simulink model "Crazyflie_NoLinealModel_EB"  (R2020b)
settings: Solver=FixedStepAuto  StartTime=0.0  StopTime=30  FixedStep=0.001  RelTol=1e-3
values from neighbouring files (symbols this model uses):
  fm = 0.2685    [Crazyflie_Model.m]
  we = sqrt((m*g)/(4*CT))    [Crazyflie_Model.m]
undefined symbols (not defined in the file or in its folder): DiscIntNeverNeededParam, Dphi_s, Dphi_T, Dpsi_s, Dtheta_s, KIz, magnitude, MCO, Phi_s, Phi_T, phi_theta_limit, quad, Theta_s, U_s, V_s, X_s, X_T, XY_delta, xyv_lim, Y_s, Yaw_delta, Yaw_s, Yaw_T, Z_delta, Z_s, Z_T
libraries: simulink x16, pid_lib x11
(part 2 of 2)

== system Crazyflie_NoLinealModel_EB/On-board Controllers/Control Mixer ==
  OMEGA : Inport
  Dpitch : Inport  Port=2
  Droll : Inport  Port=3
  Dyaw : Inport  Port=4
  Enable : EnablePort
  Demux : Demux
  Gain : Gain  Gain=MCO  Multiplication=Matrix(K*u) (u vector)
  Mux : Mux
  PWM1 : Outport
  PWM2 : Outport  Port=2
  PWM3 : Outport  Port=3
  PWM4 : Outport  Port=4
  wires:
  Mux/1 -> Gain/1
  Gain/1 -> Demux/1
  Demux/3 -> PWM3/1
  Demux/1 -> PWM1/1
  Demux/2 -> PWM2/1
  Droll/1 -> Mux/3
  OMEGA/1 -> Mux/1
  Dyaw/1 -> Mux/4
  Dpitch/1 -> Mux/2
  Demux/4 -> PWM4/1

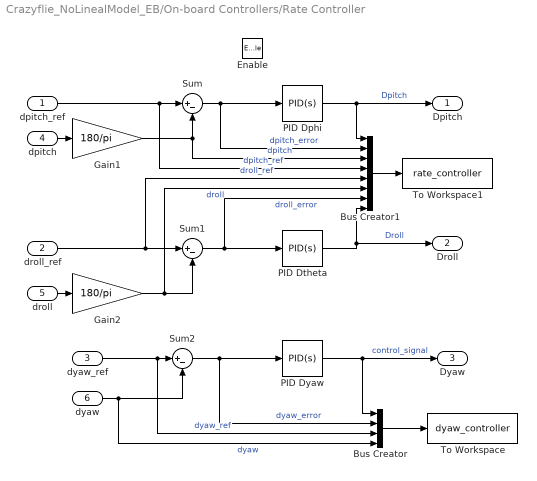
== system Crazyflie_NoLinealModel_EB/On-board Controllers/Rate Controller ==
  dpitch_ref : Inport
  droll_ref : Inport  Port=2
  dyaw_ref : Inport  Port=3
  dpitch : Inport  Port=4
  droll : Inport  Port=5
  dyaw : Inport  Port=6
  Enable : EnablePort
  Bus Creator : BusCreator  Inputs=4
  Bus Creator1 : BusCreator  Inputs=8
  Gain1 : Gain  Gain=180/pi
  Gain2 : Gain  Gain=180/pi
  PID Dphi : pid_lib/PID Controller  Controller=PID  Form=Parallel  TimeDomain=Continuous-time  UseExternalTs=off  SampleTime=-1  IntegratorMethod=Forward Euler  FilterMethod=Forward Euler  ControllerParametersSource=internal  P=Dphi_s(1)  I=Dphi_s(2)  D=Dphi_s(3)  UseFilter=on  N=100  TunerSelectOption=Transfer Function Based (PID Tuner App)  InitialConditionSource=internal  InitialConditionForIntegrator=0  InitialConditionForFilter=0  DifferentiatorICPrevScaledInput=0  ExternalReset=none  TrackingMode=off  Kt=1  LimitOutput=off  SatLimitsSource=internal  UpperSaturationLimit=inf  LowerSaturationLimit=-inf  LinearizeAsGain=on  AntiWindupMode=none  Kb=1  POutMin=[]  POutMax=[]  IOutMin=[]  IOutMax=[]  DOutMin=[]  DOutMax=[]  NOutMin=[]  NOutMax=[]  SumOutMin=[]  SumOutMax=[]  SaturationOutMin=[]  SaturationOutMax=[]  PParamMin=[]  PParamMax=[]  IParamMin=[]  IParamMax=[]  DParamMin=[]  DParamMax=[]  NParamMin=[]  NParamMax=[]  KbParamMin=[]  KbParamMax=[]  KtParamMin=[]  KtParamMax=[]  KbOutMin=[]  KbOutMax=[]  KtOutMin=[]  KtOutMax=[]  IntegratorOutMin=[]  IntegratorOutMax=[]  FilterOutMin=[]  FilterOutMax=[]  SumI1OutMin=[]  SumI1OutMax=[]  SumI2OutMin=[]  SumI2OutMax=[]  SumI3OutMin=[]  SumI3OutMax=[]  SumI4OutMin=[]  SumI4OutMax=[]  SumDOutMin=[]  SumDOutMax=[]  DifferentiatorOutMin=[]  DifferentiatorOutMax=[]  FilterDiffOutCoefMin=[]  FilterDiffOutCoefMax=[]  ReciprocalOutMin=[]  ReciprocalOutMax=[]  SumDenOutMin=[]  SumDenOutMax=[]  SumNumOutMin=[]  SumNumOutMax=[]  DivideOutMin=[]  DivideOutMax=[]  UdiffTsProdOutMin=[]  UdiffTsProdOutMax=[]  NTsProdOutMin=[]  NTsProdOutMax=[]  UintegralTsProdOutMin=[]  UintegralTsProdOutMax=[]  UngainTsProdOutMin=[]  UngainTsProdOutMax=[]  IntegratorContinuousStateAttributes=''  IntegratorStateMustResolveToSignalObject=off  IntegratorRTWStateStorageClass=Auto  FilterContinuousStateAttributes=''  FilterStateMustResolveToSignalObject=off  FilterRTWStateStorageClass=Auto  ParallelPVariant=InternalParameters  IdealPVariant=Disabled  IVariant=InternalParameters  DVariant=InternalParameters  IntegratorVariant=Continuous  SatVariant=Disabled  AWVariant=Passthrough  PCopyVariant=Disabled  TRVariant=Disabled  FdbkBlocksVariant=Forward  IdealPFdbkVariant=Disabled  SatFdbkVariant=Disabled  DerivativeFilterVariant=ContFilter  NVariant=InternalParameters  NCopyVariant=Disabled  FilterICVariant=InternalICsFilter  IntegratorICVariant=InternalICs  ExternalResetVariant=Disabled  TRSumVariant=Passthrough  SumFdbkVariant=Disabled  SumVariant=Sum_PID  TsampFilterVariant=InternalTs  TsampNgainVariant=Passthrough  TsampIntegralVariant=Passthrough  ExternalSaturationOutDataTypeStr=Inherit: Same as second input
  PID Dtheta : pid_lib/PID Controller  Controller=PID  Form=Parallel  TimeDomain=Continuous-time  UseExternalTs=off  SampleTime=-1  IntegratorMethod=Forward Euler  FilterMethod=Forward Euler  ControllerParametersSource=internal  P=Dtheta_s(1)  I=Dtheta_s(2)  D=Dtheta_s(3)  UseFilter=on  N=100  TunerSelectOption=Transfer Function Based (PID Tuner App)  InitialConditionSource=internal  InitialConditionForIntegrator=0  InitialConditionForFilter=0  DifferentiatorICPrevScaledInput=0  ExternalReset=none  TrackingMode=off  Kt=1  LimitOutput=off  SatLimitsSource=internal  UpperSaturationLimit=inf  LowerSaturationLimit=-inf  LinearizeAsGain=on  AntiWindupMode=none  Kb=1  POutMin=[]  POutMax=[]  IOutMin=[]  IOutMax=[]  DOutMin=[]  DOutMax=[]  NOutMin=[]  NOutMax=[]  SumOutMin=[]  SumOutMax=[]  SaturationOutMin=[]  SaturationOutMax=[]  PParamMin=[]  PParamMax=[]  IParamMin=[]  IParamMax=[]  DParamMin=[]  DParamMax=[]  NParamMin=[]  NParamMax=[]  KbParamMin=[]  KbParamMax=[]  KtParamMin=[]  KtParamMax=[]  KbOutMin=[]  KbOutMax=[]  KtOutMin=[]  KtOutMax=[]  IntegratorOutMin=[]  IntegratorOutMax=[]  FilterOutMin=[]  FilterOutMax=[]  SumI1OutMin=[]  SumI1OutMax=[]  SumI2OutMin=[]  SumI2OutMax=[]  SumI3OutMin=[]  SumI3OutMax=[]  SumI4OutMin=[]  SumI4OutMax=[]  SumDOutMin=[]  SumDOutMax=[]  DifferentiatorOutMin=[]  DifferentiatorOutMax=[]  FilterDiffOutCoefMin=[]  FilterDiffOutCoefMax=[]  ReciprocalOutMin=[]  ReciprocalOutMax=[]  SumDenOutMin=[]  SumDenOutMax=[]  SumNumOutMin=[]  SumNumOutMax=[]  DivideOutMin=[]  DivideOutMax=[]  UdiffTsProdOutMin=[]  UdiffTsProdOutMax=[]  NTsProdOutMin=[]  NTsProdOutMax=[]  UintegralTsProdOutMin=[]  UintegralTsProdOutMax=[]  UngainTsProdOutMin=[]  UngainTsProdOutMax=[]  IntegratorContinuousStateAttributes=''  IntegratorStateMustResolveToSignalObject=off  IntegratorRTWStateStorageClass=Auto  FilterContinuousStateAttributes=''  FilterStateMustResolveToSignalObject=off  FilterRTWStateStorageClass=Auto  ParallelPVariant=InternalParameters  IdealPVariant=Disabled  IVariant=InternalParameters  DVariant=InternalParameters  IntegratorVariant=Continuous  SatVariant=Disabled  AWVariant=Passthrough  PCopyVariant=Disabled  TRVariant=Disabled  FdbkBlocksVariant=Forward  IdealPFdbkVariant=Disabled  SatFdbkVariant=Disabled  DerivativeFilterVariant=ContFilter  NVariant=InternalParameters  NCopyVariant=Disabled  FilterICVariant=InternalICsFilter  IntegratorICVariant=InternalICs  ExternalResetVariant=Disabled  TRSumVariant=Passthrough  SumFdbkVariant=Disabled  SumVariant=Sum_PID  TsampFilterVariant=InternalTs  TsampNgainVariant=Passthrough  TsampIntegralVariant=Passthrough  ExternalSaturationOutDataTypeStr=Inherit: Same as second input
  PID Dyaw : pid_lib/PID Controller  Controller=PID  Form=Parallel  TimeDomain=Continuous-time  UseExternalTs=off  SampleTime=-1  IntegratorMethod=Forward Euler  FilterMethod=Forward Euler  ControllerParametersSource=internal  P=Dpsi_s(1)  I=Dpsi_s(2)  D=Dpsi_s(3)  UseFilter=on  N=100  TunerSelectOption=Transfer Function Based (PID Tuner App)  InitialConditionSource=internal  InitialConditionForIntegrator=0  InitialConditionForFilter=0  DifferentiatorICPrevScaledInput=0  ExternalReset=none  TrackingMode=off  Kt=1  LimitOutput=off  SatLimitsSource=internal  UpperSaturationLimit=inf  LowerSaturationLimit=-inf  LinearizeAsGain=on  AntiWindupMode=none  Kb=1  POutMin=[]  POutMax=[]  IOutMin=[]  IOutMax=[]  DOutMin=[]  DOutMax=[]  NOutMin=[]  NOutMax=[]  SumOutMin=[]  SumOutMax=[]  SaturationOutMin=[]  SaturationOutMax=[]  PParamMin=[]  PParamMax=[]  IParamMin=[]  IParamMax=[]  DParamMin=[]  DParamMax=[]  NParamMin=[]  NParamMax=[]  KbParamMin=[]  KbParamMax=[]  KtParamMin=[]  KtParamMax=[]  KbOutMin=[]  KbOutMax=[]  KtOutMin=[]  KtOutMax=[]  IntegratorOutMin=[]  IntegratorOutMax=[]  FilterOutMin=[]  FilterOutMax=[]  SumI1OutMin=[]  SumI1OutMax=[]  SumI2OutMin=[]  SumI2OutMax=[]  SumI3OutMin=[]  SumI3OutMax=[]  SumI4OutMin=[]  SumI4OutMax=[]  SumDOutMin=[]  SumDOutMax=[]  DifferentiatorOutMin=[]  DifferentiatorOutMax=[]  FilterDiffOutCoefMin=[]  FilterDiffOutCoefMax=[]  ReciprocalOutMin=[]  ReciprocalOutMax=[]  SumDenOutMin=[]  SumDenOutMax=[]  SumNumOutMin=[]  SumNumOutMax=[]  DivideOutMin=[]  DivideOutMax=[]  UdiffTsProdOutMin=[]  UdiffTsProdOutMax=[]  NTsProdOutMin=[]  NTsProdOutMax=[]  UintegralTsProdOutMin=[]  UintegralTsProdOutMax=[]  UngainTsProdOutMin=[]  UngainTsProdOutMax=[]  IntegratorContinuousStateAttributes=''  IntegratorStateMustResolveToSignalObject=off  IntegratorRTWStateStorageClass=Auto  FilterContinuousStateAttributes=''  FilterStateMustResolveToSignalObject=off  FilterRTWStateStorageClass=Auto  ParallelPVariant=InternalParameters  IdealPVariant=Disabled  IVariant=InternalParameters  DVariant=InternalParameters  IntegratorVariant=Continuous  SatVariant=Disabled  AWVariant=Passthrough  PCopyVariant=Disabled  TRVariant=Disabled  FdbkBlocksVariant=Forward  IdealPFdbkVariant=Disabled  SatFdbkVariant=Disabled  DerivativeFilterVariant=ContFilter  NVariant=InternalParameters  NCopyVariant=Disabled  FilterICVariant=InternalICsFilter  IntegratorICVariant=InternalICs  ExternalResetVariant=Disabled  TRSumVariant=Passthrough  SumFdbkVariant=Disabled  SumVariant=Sum_PID  TsampFilterVariant=InternalTs  TsampNgainVariant=Passthrough  TsampIntegralVariant=Passthrough  ExternalSaturationOutDataTypeStr=Inherit: Same as second input
  Sum : Sum  Inputs=|+-
  Sum1 : Sum  Inputs=|+-
  Sum2 : Sum  Inputs=|+-
  To Workspace : ToWorkspace  VariableName=dyaw_controller  SaveFormat=Timeseries  SampleTime=-1
  To Workspace1 : ToWorkspace  VariableName=rate_controller  SaveFormat=Timeseries  SampleTime=-1
  Dpitch : Outport
  Droll : Outport  Port=2
  Dyaw : Outport  Port=3
  wires:
  dyaw/1 -> Bus Creator/4, Sum2/2  "dyaw"
  Sum/1 -> PID Dphi/1, Bus Creator1/2  "dpitch_error"
  Bus Creator1/1 -> To Workspace1/1
  dpitch/1 -> Gain1/1
  droll/1 -> Gain2/1
  PID Dyaw/1 -> Bus Creator/1, Dyaw/1  "control_signal"
  Gain1/1 -> Bus Creator1/3, Sum/2  "dpitch"
  Gain2/1 -> Bus Creator1/6, Sum1/2  "droll"
  droll_ref/1 -> Bus Creator1/5, Sum1/1  "droll_ref"
  dyaw_ref/1 -> Bus Creator/3, Sum2/1  "dyaw_ref"
  dpitch_ref/1 -> Bus Creator1/4, Sum/1  "dpitch_ref"
  PID Dphi/1 -> Dpitch/1, Bus Creator1/1  "Dpitch"
  Sum1/1 -> PID Dtheta/1, Bus Creator1/7  "droll_error"
  Bus Creator/1 -> To Workspace/1
  Sum2/1 -> PID Dyaw/1, Bus Creator/2  "dyaw_error"
  PID Dtheta/1 -> Bus Creator1/8, Droll/1  "Droll"

== system Crazyflie_NoLinealModel_EB/Event Trigered/Subsystem3/If Action Subsystem4 ==
  In2 : Inport
  Enable : EnablePort
  Out2 : Outport
  wires:
  In2/1 -> Out2/1

== system Crazyflie_NoLinealModel_EB/Event Trigered/Subsystem4/If Action Subsystem4 ==
  In2 : Inport
  Enable : EnablePort
  Out2 : Outport
  wires:
  In2/1 -> Out2/1

== system Crazyflie_NoLinealModel_EB/Event Trigered/XY Trigger Signal/If Action Subsystem1 ==
  In2 : Inport
  Enable : EnablePort
  Out2 : Outport
  wires:
  In2/1 -> Out2/1

== system Crazyflie_NoLinealModel_EB/Event Trigered/XY Trigger Signal/If Action Subsystem2 ==
  XY_dron : Inport
  Enable : EnablePort
  Out2 : Outport
  wires:
  XY_dron/1 -> Out2/1

== system Crazyflie_NoLinealModel_EB/Event Trigered/Yaw Trigger Signal/If Action Subsystem2 ==
  yaw_dron : Inport
  Enable : EnablePort
  Out2 : Outport
  wires:
  yaw_dron/1 -> Out2/1

== system Crazyflie_NoLinealModel_EB/Event Trigered/Yaw Trigger Signal/If Action Subsystem3 ==
  In2 : Inport
  Enable : EnablePort
  Out2 : Outport
  wires:
  In2/1 -> Out2/1

== system Crazyflie_NoLinealModel_EB/Event Trigered/Z Trigger Signal/If Action Subsystem1 ==
  In2 : Inport
  Enable : EnablePort
  Out2 : Outport
  wires:
  In2/1 -> Out2/1

== system Crazyflie_NoLinealModel_EB/Event Trigered/Z Trigger Signal/If Action Subsystem2 ==
  Z_dron : Inport
  Enable : EnablePort
  Out2 : Outport
  wires:
  Z_dron/1 -> Out2/1

== matlab function Crazyflie_NoLinealModel_EB/Crazyflie2.0  Non-Linear Model/MATLAB Function ==
  data: uvw input; xyz_dot output; angles input
function xyz_dot  = Position(uvw,angles)
xyz_dot = zeros(3,1);
phi = angles(1); %*pi/180;
theta = angles(2); %*pi/180;
psi = angles(3); %*pi/180;
Tb_o = [cos(theta)*cos(psi)                                cos(theta)*sin(psi)                             -sin(theta)  ;   %BBF > Inertial rotation matrix
        sin(phi)*sin(theta)*cos(psi)-cos(phi)*sin(psi)    sin(phi)*sin(theta)*sin(psi)+cos(phi)*cos(psi)  sin(phi)*cos(theta) ;
        cos(phi)*sin(theta)*cos(psi)+sin(phi)*sin(psi)    cos(phi)*sin(theta)*sin(psi)-sin(phi)*cos(psi)   cos(phi)*cos(theta)];

xyz_dot = (Tb_o')*uvw;
end

== matlab function Crazyflie_NoLinealModel_EB/Off-board Controllers [100Hz]/X-Y Controller/Error to Body Frame ==
  data: xc input; xbe output; yc input; x input; y input; psi input; ybe output
function [xbe, ybe] = fcn(xc, yc, x, y, psi)

xe = xc-x;
ye = yc-y;

xbe = xe*cos(psi)+ye*sin(psi);
ybe = -xe*sin(psi)+ye*cos(psi);

== matlab function Crazyflie_NoLinealModel_EB/Crazyflie2.0  Non-Linear Model/MATLAB Function1 ==
  data: pqr input; angles_dot output; angles input
function angles_dot  = Angle(pqr,angles)
angles_dot = zeros(3,1);
phi = angles(1); %*pi/180;
theta = angles(2); %*pi/180;

H = [1    sin(phi)*tan(theta)     cos(phi)*tan(theta)
     0       cos(phi)                 -sin(phi)   
     0       sin(phi)/cos(theta)    cos(phi)/cos(theta)];
angles_dot = H*pqr;
end

== matlab function Crazyflie_NoLinealModel_EB/Crazyflie2.0  Non-Linear Model/MATLAB Function2 ==
  data: uvw input; uvw_dot output; pqr input; angles input; F input
function uvw_dot  = Forces(uvw,pqr,angles,F)
uvw_dot = zeros(3,1);
Force = [0;0;F];
g_o = [0;0;-9.81];
phi = angles(1); %*pi/180;
theta = angles(2); %*pi/180;
psi = angles(3); %*pi/180;
Rx = [1 0 0; 0 cos(phi) sin(phi); 0 -sin(phi) cos(phi)];
Ry = [cos(theta) 0 -sin(theta); 0 1 0; sin(theta) 0 cos(theta)];
Rz = [cos(psi) sin(psi) 0; -sin(psi) cos(psi) 0; 0 0 1];
Tb_o = Rx*Ry*Rz;
% Tb_o = [cos(theta)*cos(psi)                                cos(theta)*sin(psi)                             -sin(theta)  ;   %BBF > Inertial rotation matrix
%         sin(phi)*sin(theta)*cos(psi)-cos(phi)*sin(psi)    sin(phi)*sin(theta)*sin(psi)+cos(phi)*cos(psi)  sin(phi)*cos(theta) ;
%         cos(phi)*sin(theta)*cos(psi)+sin(phi)*sin(psi)    cos(phi)*sin(theta)*sin(psi)-sin(phi)*cos(psi)   cos(phi)*cos(theta)];

    uvw_dot = Force + Tb_o*g_o - cross(pqr,uvw);

end

== matlab function Crazyflie_NoLinealModel_EB/Crazyflie2.0  Non-Linear Model/MATLAB Function3 ==
  data: pqr_dot output; pqr input; M input
function pqr_dot  = Moments(pqr,M)
pqr_dot = zeros(3,1);
Ixx =  1.395e-05;  %2.3951e-5; %1.39e-05; %2.51943e-5; % % %
Iyy = 1.436e-05; %2.3951e-5; %1.436e-05; % 2.54379e-5; % %         %
Izz =  2.173e-05;  %3.2347e-5; %2.173e-05 ; %4.51407e-5; % %         %;%0.160;
J = diag([Ixx Iyy Izz]);    %   I  Flyer rotational inertia matrix     3x3
pqr_dot = inv(J)*(M-cross(pqr,J*pqr));
end
